simulink model "NLDP"  (R2022b)
settings: Solver=VariableStepAuto  StartTime=0.0  StopTime=70  RelTol=1e-3
values from neighbouring files (symbols this model uses):
  c = 0.25    [NLDP.m]
  g = 9.81    [NLDP.m]
  L = 2.0    (= 2)    [NLDP.m]
  m = 1.0    (= 1)    [NLDP.m]
settings Model: Creator=sooru  LastModifiedBy=sooru

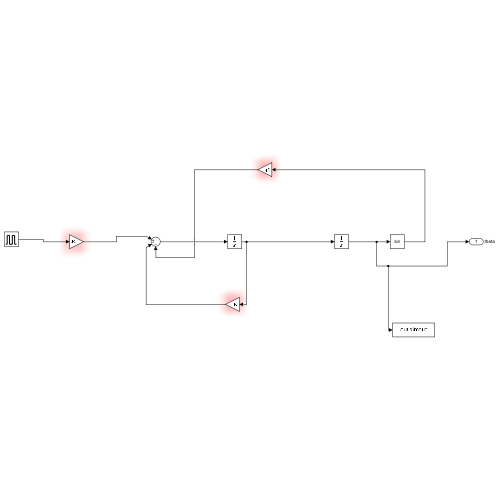
[thumbnail: Simulink's stored preview of the top-level diagram]
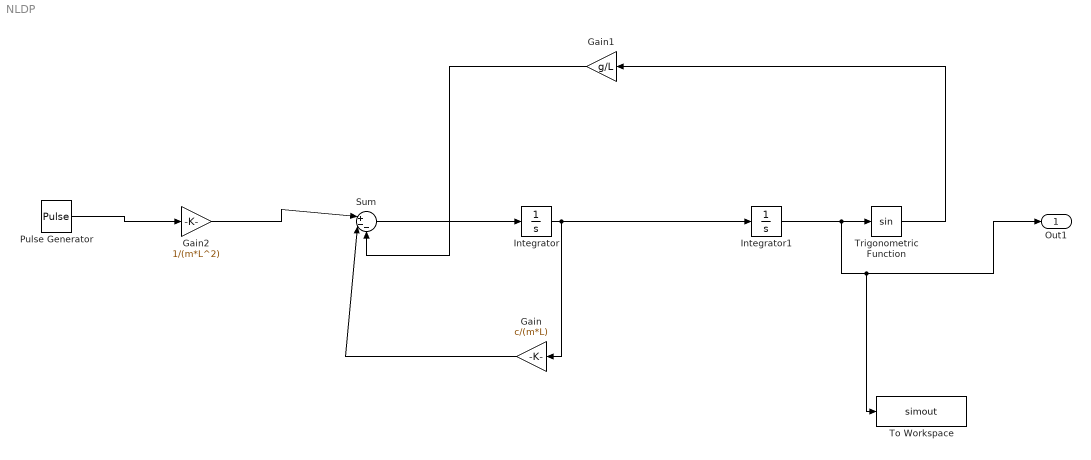
== system NLDP ==
  Gain : Gain  Gain=c/(m*L)
  Gain1 : Gain  Gain=g/L
  Gain2 : Gain  Gain=1/(m*L^2)
  Integrator : Integrator
  Integrator1 : Integrator
  Pulse Generator : DiscretePulseGenerator  PulseType=Time based  Amplitude=10  Period=100  PulseWidth=2
  Sum : Sum  Inputs=|+--
  To Workspace : ToWorkspace  VariableName=simout  SaveFormat=Timeseries  SampleTime=-1
  Trigonometric Function : Trigonometry
  Out1 : Outport  SignalName=theta
  wires:
  Integrator/1 -> Gain/1, Integrator1/1
  Pulse Generator/1 -> Gain2/1
  Gain2/1 -> Sum/1
  Gain/1 -> Sum/2
  Sum/1 -> Integrator/1
  Gain1/1 -> Sum/3
  Integrator1/1 -> Trigonometric Function/1, To Workspace/1, Out1/1
  Trigonometric Function/1 -> Gain1/1
